simulink model "VSI"  (R2018b)
settings: Solver=FixedStepDiscrete  StartTime=0.0  StopTime=inf  FixedStep=0.01  RelTol=1e-3
PostLoadFcn:
  | if any(exist('dsrtsu_mdlpostloadfcn', 'file') ~= 0), dsrtsu_mdlpostloadfcn('Execute', bdroot); end
values from neighbouring files (symbols this model uses):
  d_WheelBase = 2.8    [VSI_Local.sldd]
  P_tARawFilt = 0.2    [VSI_Local.sldd]
  P_tAxsFilt = 0.2    [VSI_Local.sldd]
  P_tSasFilt = 0.25    [VSI_Local.sldd]
  P_tVVehFilt = 0.3    [VSI_Local.sldd]
  P_tYrsFilt = 0.25    [VSI_Local.sldd]
  P_vHi = 3.0    [VSI_Local.sldd]
  P_vLo = 1.0    [VSI_Local.sldd]
  StRatio = 15.2    [VSI_Local.sldd]
libraries: LPFilter x5
settings Model: DSRTSU_INTERNAL_RTI_VER=540  DSRTSU_INTERNAL_RTI_TYPE=rti1401  RTICANMMDATA=struct('GeneralSetupData',struct('modelroot','F:\DatabaseZO\08.Code\Model\ZOP_Integration','generalsettings',struct('filesettings',struct('destfolder',struct('Name','RTICANMM_FILES','Check',1),'buildfolder',struct('Name','.','Check',1),'AbsDestfolder',struct('Name','F:\DatabaseZO\08.Code\Model\ZOP_Integration\RTICANMM_FILES'),'AbsBuildfolder',struct('Name','F:\DatabaseZO\08.Code\Model\ZOP_Integration'))),'options',struct('addpaths',1,'rmpaths',1,'addtrcexclusion',logical(1),'cannavigator',struct('checkmonitoring',0),'show_usrtrc',0,'use_usrtrc',0),'advanced',struct('options',ones(1,100)),'MPSetup',{{}},'RTI',struct('Type','RTI1401','Ver','7.12','Date','02-May-2019'),'modelname','VSI','block','VSI'))  DSRTSU_INTERNAL_RTIFPGA=130  Creator=Administrator  LastModifiedBy=zjw
settings OptimizationCC: BlockReduction=off  ConditionallyExecuteInputs=off  OptimizeBlockIOStorage=off  BufferReuse=off  GlobalBufferReuse=off  ExpressionFolding=off  PassReuseOutputArgsThreshold=0  LocalBlockOutputs=off  OptimizeBlockOrder=speed  OptimizeDataStoreBuffers=off  BusAssignmentInplaceUpdate=off
settings DebuggingCC: ParameterTunabilityLossMsg=error
settings HardwareCC: ProdBitPerPointer=32  ProdBitPerSizeT=32  ProdBitPerPtrDiffT=32  ProdLargestAtomicInteger=Integer  ProdEndianess=BigEndian  ProdWordSize=32  ProdHWDeviceType=Custom Processor->Custom  TargetIntDivRoundTo=Zero  TargetEndianess=BigEndian  TargetHWDeviceType=Custom Processor->Custom
settings ModelReferenceCC: ModelReferenceNumInstancesAllowed=Single
settings SFSimCC: MATLABDynamicMemAlloc=off
settings RTWCC: SystemTargetFile=rti1401.tlc  MakeCommand=make_rti  TemplateMakefile=rti1401.tmf  Description=dSPACE DS1401 Hardware Platform  GenerateReport=on  LaunchReport=on
settings CodeAppCC: OperatorAnnotations=on
settings STFCustomTargetCC: ParMdlRefBuildCompliant=on  SystemTargetFile=rti1401.tlc
settings GRTTargetCC: TargetLangStandard=C89/C90 (ANSI)  CompOptLevelCompliant=off  ConcurrentExecutionCompliant=off  CombineOutputUpdateFcns=off  MatFileLogging=off  CPPClassGenCompliant=off  UseToolchainInfoCompliant=off

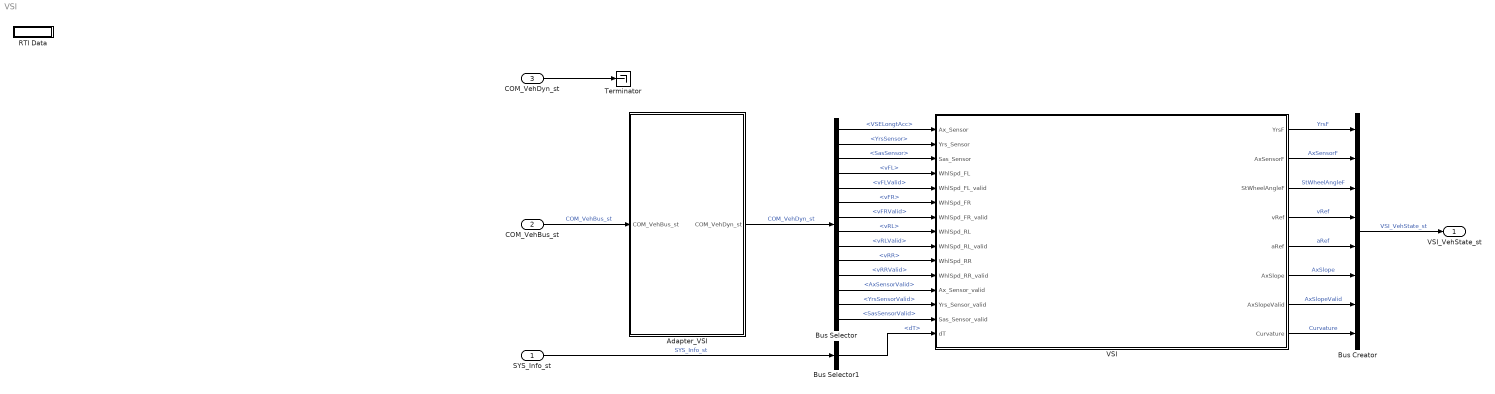
== system VSI ==
  SYS_Info_st : Inport  OutDataTypeStr=Bus: SYS_INFO_ST  BusOutputAsStruct=on
  COM_VehBus_st : Inport  Port=2  OutDataTypeStr=Bus: COM_VEHBUS_ST  BusOutputAsStruct=on
  COM_VehDyn_st : Inport  Port=3  OutDataTypeStr=Bus: COM_VEHDYN_ST  BusOutputAsStruct=on
  Adapter_VSI : Subsystem
  Bus Creator : BusCreator  Inputs=8  OutDataTypeStr=Bus: VSI_VEHSTATE_ST  NonVirtualBus=on
      settings: InheritFromInputs=off
  Bus Selector : BusSelector  OutputSignals=VSELongtAcc,YrsSensor,SasSensor,vFL,vFLValid,vFR,vFRValid,vRL,vRLValid,vRR,vRRValid,AxSensorValid,YrsSensorValid,SasSensorValid
  Bus Selector1 : BusSelector  OutputSignals=dT
  RTI Data : Subsystem  Tag=struct('RTIDataServer',struct('RTIDataServerVs','2','RTIModelDescription','struct(''main'',''VSI'',''sub'','''',''isMp'',0)'))  LoadFcn="if exist('rtidc'), try,  rtidc('DataHostBlockClbLoad', gcbh); catch, disp(['Warning: ''LoadFcn'' for RTI Data block failed: ' lasterr]); end, end,"  mask(RTI_DATA_HOST){}
      mask help:
      | RTI Data Block.
      | This block is used by RTI to store internal model-dependent data.
      | Please keep this block on the root level of the model. Deleting this block will result in data loss.
      |
      | NEVER DELETE OR COPY THIS BLOCK!
      settings: CopyFcn="if exist('rtidc'), try,  rtidc('DataHostBlockClbCopy', gcbh); catch, disp(['Warning: ''CopyFcn'' for RTI Data block failed: ' lasterr]); end, end,"  DeleteFcn="if exist('rtidc'), try,  rtidc('DataHostBlockClbDelete', gcbh); catch, disp(['Warning: ''DeleteFcn'' for RTI Data block failed: ' lasterr]); end, end,"  ModelCloseFcn="if exist('rtidc'), try,  rtidc('DataHostBlockClbModelClose', gcbh); catch, disp(['Warning: ''ModelCloseFcn'' for RTI Data block failed: ' lasterr]); end, end,"  PreSaveFcn="if exist('rtidc'), try,  rtidc('DataHostBlockClbPreSave', gcbh); catch, disp(['Warning: ''PreSaveFcn'' for RTI Data block failed: ' lasterr]); end, end,"  PostSaveFcn="if exist('rtidc'), try,  rtidc('DataHostBlockClbPostSave', gcbh); catch, disp(['Warning: ''PostSaveFcn'' for RTI Data block failed: ' lasterr]); end, end,"  NameChangeFcn="if exist('rtidc'), try,  rtidc('DataHostBlockClbNameChange', gcbh); catch, disp(['Warning: ''NameChangeFcn'' for RTI Data block failed: ' lasterr]); end, end,"
      mask Help:
      | RTI Data Block.
      | This block is used by RTI to store internal model-dependent data.
      | Please keep this block on the root level of the model. Deleting this block will result in data loss.
      | 
      | NEVER DELETE OR COPY THIS BLOCK!
      mask Display:
      | text(0.5, 0.5, 'RTI Data', 'HorizontalAlignment', 'center');
      | plot([1 0]);
  Terminator : Terminator
  VSI : Subsystem
  VSI_VehState_st : Outport  OutDataTypeStr=Bus: VSI_VEHSTATE_ST
  wires:
  Bus Selector/2 -> VSI/2(Yrs_Sensor)  "<YrsSensor>"
  Bus Selector/3 -> VSI/3(Sas_Sensor)  "<SasSensor>"
  Bus Selector/4 -> VSI/4(WhlSpd_FL)  "<vFL>"
  Bus Selector/5 -> VSI/5(WhlSpd_FL_valid)  "<vFLValid>"
  Bus Selector/6 -> VSI/6(WhlSpd_FR)  "<vFR>"
  Bus Selector/7 -> VSI/7(WhlSpd_FR_valid)  "<vFRValid>"
  Bus Selector/8 -> VSI/8(WhlSpd_RL)  "<vRL>"
  Bus Selector/9 -> VSI/9(WhlSpd_RL_valid)  "<vRLValid>"
  Bus Selector/10 -> VSI/10(WhlSpd_RR)  "<vRR>"
  Bus Selector/11 -> VSI/11(WhlSpd_RR_valid)  "<vRRValid>"
  Bus Selector/14 -> VSI/14(Sas_Sensor_valid)  "<SasSensorValid>"
  Bus Creator/1 -> VSI_VehState_st/1  "VSI_VehState_st"
  VSI/2(AxSensorF) -> Bus Creator/2  "AxSensorF"
  VSI/3(StWheelAngleF) -> Bus Creator/3  "StWheelAngleF"
  VSI/4(vRef) -> Bus Creator/4  "vRef"
  VSI/5(aRef) -> Bus Creator/5  "aRef"
  VSI/6(AxSlope) -> Bus Creator/6  "AxSlope"
  VSI/1(YrsF) -> Bus Creator/1  "YrsF"
  VSI/7(AxSlopeValid) -> Bus Creator/7  "AxSlopeValid"
  VSI/8(Curvature) -> Bus Creator/8  "Curvature"
  Bus Selector/12 -> VSI/12(Ax_Sensor_valid)  "<AxSensorValid>"
  Bus Selector/13 -> VSI/13(Yrs_Sensor_valid)  "<YrsSensorValid>"
  SYS_Info_st/1 -> Bus Selector1/1  "SYS_Info_st"
  Bus Selector1/1 -> VSI/15(dT)  "<dT>"
  COM_VehBus_st/1 -> Adapter_VSI/1(COM_VehBus_st)  "COM_VehBus_st"
  Bus Selector/1 -> VSI/1(Ax_Sensor)  "<VSELongtAcc>"
  Adapter_VSI/1(COM_VehDyn_st) -> Bus Selector/1  "COM_VehDyn_st"
  COM_VehDyn_st/1 -> Terminator/1

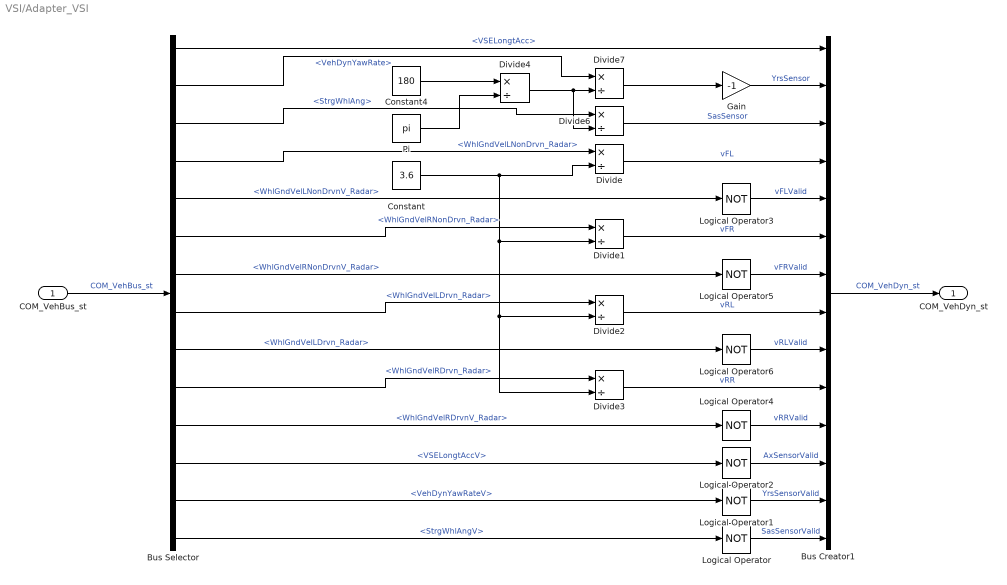
== system VSI/Adapter_VSI ==
  COM_VehBus_st : Inport  OutDataTypeStr=Bus: COM_VEHBUS_ST
  Bus Creator1 : BusCreator  Inputs=14  OutDataTypeStr=Bus: COM_VEHDYN_ST  NonVirtualBus=on
  Bus Selector : BusSelector  OutputSignals=x185.VSELongtAcc,x1E9.VehDynYawRate,x1E5.StrgWhlAng,x24E.WhlGndVelLNonDrvn_Radar,x24E.WhlGndVelLNonDrvnV_Radar,x24E.WhlGndVelRNonDrvn_Radar,x24E.WhlGndVelRNonDrvnV_Radar,x24C.WhlGndVelLDrvn_Radar,x24C.WhlGndVelLDrvn_Radar,x24C.WhlGndVelRDrvn_Radar,x24C.WhlGndVelRDrvnV_Radar,x185.VSELongtAccV,x1E9.VehDynYawRateV,x1E5.StrgWhlAngV
  Constant : Constant  Value=3.6
  Constant4 : Constant  Value=180
  Divide{,1..3,6..7} (6 alike) : Product  Inputs=*/  OutDataTypeStr=single
  Divide4 : Product  Inputs=*/
  Gain : Gain  Gain=-1
  Logical Operator{,1..6} (7 alike) : Logic  Operator=NOT  AllPortsSameDT=off  OutDataTypeStr=boolean
  Pi : Constant  Value=pi  OutDataTypeStr=Inherit: Inherit via back propagation
  COM_VehDyn_st : Outport  OutDataTypeStr=Bus: COM_VEHDYN_ST
  wires:
  Divide3/1 -> Bus Creator1/10  "vRR"
  Divide4/1 -> Divide6/2, Divide7/2
  Logical Operator2/1 -> Bus Creator1/12  "AxSensorValid"
  Divide/1 -> Bus Creator1/4  "vFL"
  Logical Operator1/1 -> Bus Creator1/13  "YrsSensorValid"
  Divide7/1 -> Gain/1
  Divide6/1 -> Bus Creator1/3  "SasSensor"
  Constant4/1 -> Divide4/1
  Logical Operator5/1 -> Bus Creator1/7  "vFRValid"
  Divide1/1 -> Bus Creator1/6  "vFR"
  Logical Operator4/1 -> Bus Creator1/11  "vRRValid"
  Bus Creator1/1 -> COM_VehDyn_st/1  "COM_VehDyn_st"
  Logical Operator3/1 -> Bus Creator1/5  "vFLValid"
  Divide2/1 -> Bus Creator1/8  "vRL"
  Logical Operator6/1 -> Bus Creator1/9  "vRLValid"
  Constant/1 -> Divide3/2, Divide2/2, Divide1/2, Divide/2
  Logical Operator/1 -> Bus Creator1/14  "SasSensorValid"
  COM_VehBus_st/1 -> Bus Selector/1  "COM_VehBus_st"
  Bus Selector/1 -> Bus Creator1/1  "<VSELongtAcc>"
  Pi/1 -> Divide4/2
  Bus Selector/2 -> Divide7/1  "<VehDynYawRate>"
  Bus Selector/5 -> Logical Operator3/1  "<WhlGndVelLNonDrvnV_Radar>"
  Bus Selector/7 -> Logical Operator5/1  "<WhlGndVelRNonDrvnV_Radar>"
  Bus Selector/9 -> Logical Operator6/1  "<WhlGndVelLDrvn_Radar>"
  Bus Selector/11 -> Logical Operator4/1  "<WhlGndVelRDrvnV_Radar>"
  Bus Selector/12 -> Logical Operator2/1  "<VSELongtAccV>"
  Bus Selector/13 -> Logical Operator1/1  "<VehDynYawRateV>"
  Bus Selector/14 -> Logical Operator/1  "<StrgWhlAngV>"
  Bus Selector/4 -> Divide/1  "<WhlGndVelLNonDrvn_Radar>"
  Bus Selector/6 -> Divide1/1  "<WhlGndVelRNonDrvn_Radar>"
  Bus Selector/8 -> Divide2/1  "<WhlGndVelLDrvn_Radar>"
  Bus Selector/10 -> Divide3/1  "<WhlGndVelRDrvn_Radar>"
  Bus Selector/3 -> Divide6/1  "<StrgWhlAng>"
  Gain/1 -> Bus Creator1/2  "YrsSensor"

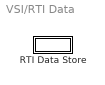
== system VSI/RTI Data ==
  RTI Data Store : Subsystem  Tag="struct('private',struct('version',struct('dsVer',uint32(2),'dsVerCreation',uint32(2),'RTI',struct('ver','7.12','type','RTI1401')),'access',struct('type','Model','isPerm',1,'created',['20-Nov-2020 11:10:38'],'modified',['07-Jan-2021 20:09:42'],'location','')),'public',struct('main',struct('data',[]),'sub',struct('name',{{'VSI'}},'data',{{struct('TH',struct('thTaskInfo',struct('taskType',{'TIMER','HWINT','TMRINT','SWINT','GLINT'},'tasksNumOf',{1,0,0,0,0},'srcIds',{{'TIMERA'},{},{},{},{}},'taskNames',{{['Timer Task 1']},{},{},{},{}})),'th_tc',struct('dataType','TASK','taskGroupId','','taskGroupList',{{}},'taskSchedulingPolicy','FCFS','taskType','TIMER','blkh',-1,'srcId','TIMERA','srcSgnName',['Timer A interrupt'],'srcCpuName','','taskName',['Timer Task 1  [0.01] s'],'taskNameDisplayExt','','smplTime',0.01,'smplTimeOffs',0,'hasFixedPriority',0,'priority',1,'hasFixedOvc',0,'ovcType',1,'ovcMax',1),'tc_th',struct('dataType','TASK','taskGroupId','','taskGroupList',{{}},'taskSchedulingPolicy','FCFS','taskType','TIMER','blkh',-1,'srcId','TIMERA','srcSgnName',['Timer A interrupt'],'srcCpuName','','taskName',['Timer Task 1  [0.01] s'],'taskNameDisplayExt','','smplTime',0.01,'smplTimeOffs',0,'hasFixedPriority',0,'priority',1,'hasFixedOvc',0,'ovcType',3,'ovcMax',1))}})))"  mask(RTI_DATA_STORE){}
      mask help:
      | RTI Data Store Block. This block is used by RTI to store internal model dependent data. Deleting this block will result in data loss.
      |
      | NEVER DELETE, COPY, OR MODIFY THIS BLOCK!
      mask Help:
      | RTI Data Store Block. This block is used by RTI to store internal model dependent data. Deleting this block will result in data loss.
      | 
      | NEVER DELETE, COPY, OR MODIFY THIS BLOCK!
      mask Display: text(0.5, 0.5, ' ', 'HorizontalAlignment', 'center');

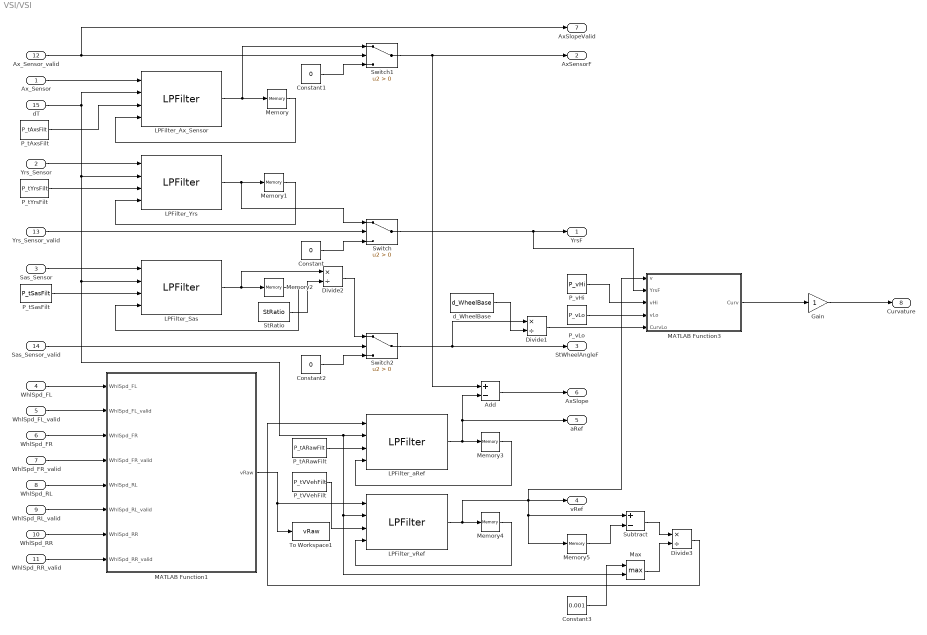
== system VSI/VSI ==
  Ax_Sensor : Inport
  Yrs_Sensor : Inport  Port=2
  Sas_Sensor : Inport  Port=3
  WhlSpd_FL : Inport  Port=4
  WhlSpd_FL_valid : Inport  Port=5
  WhlSpd_FR : Inport  Port=6
  WhlSpd_FR_valid : Inport  Port=7
  WhlSpd_RL : Inport  Port=8
  WhlSpd_RL_valid : Inport  Port=9
  WhlSpd_RR : Inport  Port=10
  WhlSpd_RR_valid : Inport  Port=11
  Ax_Sensor_valid : Inport  Port=12
  Yrs_Sensor_valid : Inport  Port=13
  Sas_Sensor_valid : Inport  Port=14
  dT : Inport  Port=15
  Add : Sum  Inputs=+-
  Constant : Constant  Value=0
  Constant1 : Constant  Value=0
  Constant2 : Constant  Value=0
  Constant3 : Constant  Value=0.001
  Divide1 : Product  Inputs=*/
  Divide2 : Product  Inputs=*/
  Divide3 : Product  Inputs=*/
  Gain : Gain
  LPFilter_Ax_Sensor : LPFilter/LPFilter  SystemSampleTime=-1
      settings: SourceProductName=CustomLib
  LPFilter_Sas : LPFilter/LPFilter  SystemSampleTime=-1
      settings: SourceProductName=CustomLib
  LPFilter_Yrs : LPFilter/LPFilter  SystemSampleTime=-1
      settings: SourceProductName=CustomLib
  LPFilter_aRef : LPFilter/LPFilter  SystemSampleTime=-1
      settings: SourceProductName=CustomLib
  LPFilter_vRef : LPFilter/LPFilter  SystemSampleTime=-1
      settings: SourceProductName=CustomLib
  MATLAB Function1 : MATLAB Function  TreatAsAtomicUnit=on
  MATLAB Function3 : MATLAB Function  TreatAsAtomicUnit=on
  Max : MinMax  Function=max  Inputs=2  OutDataTypeStr=single
  Memory{,1..5} (6 alike) : Memory
  P_tARawFilt : Constant  Value=P_tARawFilt
  P_tAxsFilt : Constant  Value=P_tAxsFilt
  P_tSasFilt : Constant  Value=P_tSasFilt
  P_tVVehFilt : Constant  Value=P_tVVehFilt
  P_tYrsFilt : Constant  Value=P_tYrsFilt
  P_vHi : Constant  Value=P_vHi
  P_vLo : Constant  Value=P_vLo
  StRatio : Constant  Value=StRatio
  Subtract : Sum  Inputs=+-
  Switch : Switch  Criteria=u2 > Threshold  OutDataTypeStr=single
  Switch1 : Switch  Criteria=u2 > Threshold  OutDataTypeStr=single
  Switch2 : Switch  Criteria=u2 > Threshold
  To Workspace1 : ToWorkspace  VariableName=vRaw  SaveFormat=Timeseries  SampleTime=-1
  d_WheelBase : Constant  Value=d_WheelBase
  YrsF : Outport
  AxSensorF : Outport  Port=2
  StWheelAngleF : Outport  Port=3
  vRef : Outport  Port=4
  aRef : Outport  Port=5
  AxSlope : Outport  Port=6
  AxSlopeValid : Outport  Port=7
  Curvature : Outport  Port=8
  wires:
  Switch1/1 -> AxSensorF/1, Add/1
  LPFilter_aRef/1 -> Memory3/1, aRef/1, Add/2
  Switch2/1 -> StWheelAngleF/1, Divide1/1
  WhlSpd_RR/1 -> MATLAB Function1/7(WhlSpd_RR)
  Constant2/1 -> Switch2/3
  MATLAB Function3/1(Curv) -> Gain/1
  MATLAB Function1/1(vRaw) -> To Workspace1/1, LPFilter_vRef/1
  WhlSpd_RL/1 -> MATLAB Function1/5(WhlSpd_RL)
  Switch/1 -> MATLAB Function3/2(YrsF), YrsF/1
  Constant/1 -> Switch/3
  Constant1/1 -> Switch1/3
  LPFilter_Ax_Sensor/1 -> Memory/1, Switch1/1
  P_vHi/1 -> MATLAB Function3/3(vHi)
  Ax_Sensor/1 -> LPFilter_Ax_Sensor/1
  Add/1 -> AxSlope/1
  Sas_Sensor_valid/1 -> Switch2/2
  WhlSpd_FL/1 -> MATLAB Function1/1(WhlSpd_FL)
  WhlSpd_FL_valid/1 -> MATLAB Function1/2(WhlSpd_FL_valid)
  WhlSpd_FR/1 -> MATLAB Function1/3(WhlSpd_FR)
  WhlSpd_FR_valid/1 -> MATLAB Function1/4(WhlSpd_FR_valid)
  WhlSpd_RL_valid/1 -> MATLAB Function1/6(WhlSpd_RL_valid)
  Yrs_Sensor_valid/1 -> Switch/2
  WhlSpd_RR_valid/1 -> MATLAB Function1/8(WhlSpd_RR_valid)
  Ax_Sensor_valid/1 -> AxSlopeValid/1, Switch1/2
  P_vLo/1 -> MATLAB Function3/4(vLo)
  Divide1/1 -> MATLAB Function3/5(CurvLo)
  dT/1 -> Max/2, LPFilter_vRef/2, LPFilter_aRef/2, LPFilter_Sas/2, LPFilter_Yrs/2, LPFilter_Ax_Sensor/2
  P_tAxsFilt/1 -> LPFilter_Ax_Sensor/3
  Yrs_Sensor/1 -> LPFilter_Yrs/1
  LPFilter_Yrs/1 -> Memory1/1, Switch/1
  P_tYrsFilt/1 -> LPFilter_Yrs/3
  LPFilter_Sas/1 -> Memory2/1, Divide2/1
  Sas_Sensor/1 -> LPFilter_Sas/1
  P_tSasFilt/1 -> LPFilter_Sas/3
  Divide2/1 -> Switch2/1
  StRatio/1 -> Divide2/2
  P_tARawFilt/1 -> LPFilter_aRef/3
  LPFilter_vRef/1 -> Memory4/1, MATLAB Function3/1(v), Memory5/1, Subtract/1, vRef/1
  P_tVVehFilt/1 -> LPFilter_vRef/3
  Memory5/1 -> Subtract/2
  Divide3/1 -> LPFilter_aRef/1
  Subtract/1 -> Divide3/1
  Memory3/1 -> LPFilter_aRef/4
  Memory4/1 -> LPFilter_vRef/4
  Memory/1 -> LPFilter_Ax_Sensor/4
  Memory1/1 -> LPFilter_Yrs/4
  Memory2/1 -> LPFilter_Sas/4
  Max/1 -> Divide3/2
  Constant3/1 -> Max/1
  d_WheelBase/1 -> Divide1/2
  Gain/1 -> Curvature/1

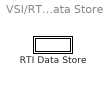
== system VSI/RTI Data/RTI Data Store ==
  RTI Data Store : Subsystem  mask(RTI_DATA_STORE){}
      mask help:
      | RTI Data Store Block. This block is used by RTI to store internal model dependent data. Deleting this block will result in data loss.
      |
      | NEVER DELETE, COPY, OR MODIFY THIS BLOCK!
      mask Help:
      | RTI Data Store Block. This block is used by RTI to store internal model dependent data. Deleting this block will result in data loss.
      | 
      | NEVER DELETE, COPY, OR MODIFY THIS BLOCK!
      mask Display: text(0.5, 0.5, ' ', 'HorizontalAlignment', 'center');

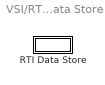
== system VSI/RTI Data/RTI Data Store/RTI Data Store ==
  RTI Data Store : Subsystem  mask(RTI_DATA_STORE){}
      mask help:
      | RTI Data Store Block. This block is used by RTI to store internal model dependent data. Deleting this block will result in data loss.
      |
      | NEVER DELETE, COPY, OR MODIFY THIS BLOCK!
      mask Help:
      | RTI Data Store Block. This block is used by RTI to store internal model dependent data. Deleting this block will result in data loss.
      | 
      | NEVER DELETE, COPY, OR MODIFY THIS BLOCK!
      mask Display: text(0.5, 0.5, ' ', 'HorizontalAlignment', 'center');

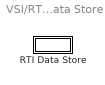
== system VSI/RTI Data/RTI Data Store/RTI Data Store/RTI Data Store ==
  RTI Data Store : Subsystem  mask(RTI_DATA_STORE){}
      mask help:
      | RTI Data Store Block. This block is used by RTI to store internal model dependent data. Deleting this block will result in data loss.
      |
      | NEVER DELETE, COPY, OR MODIFY THIS BLOCK!
      mask Help:
      | RTI Data Store Block. This block is used by RTI to store internal model dependent data. Deleting this block will result in data loss.
      | 
      | NEVER DELETE, COPY, OR MODIFY THIS BLOCK!
      mask Display: text(0.5, 0.5, ' ', 'HorizontalAlignment', 'center');

== system VSI/RTI Data/RTI Data Store/RTI Data Store/RTI Data Store/RTI Data Store ==

== matlab function VSI/MATLAB Function1 ==
  data: WhlSpd_FL input; WhlSpd_FL_valid input; WhlSpd_FR input; WhlSpd_FR_valid input; WhlSpd_RL input; WhlSpd_RL_valid input; WhlSpd_RR input; WhlSpd_RR_valid input; vRaw output
function vRaw = vRef_cal(WhlSpd_FL,WhlSpd_FL_valid,WhlSpd_FR,WhlSpd_FR_valid,WhlSpd_RL,WhlSpd_RL_valid,WhlSpd_RR,WhlSpd_RR_valid)

WhlSpd_valid_cnt = 0;
if (WhlSpd_FL_valid)
    WhlSpd_valid_cnt = WhlSpd_valid_cnt + 1;
else
end
if (WhlSpd_FR_valid)
    WhlSpd_valid_cnt = WhlSpd_valid_cnt + 1;
else
end
if (WhlSpd_RL_valid)
    WhlSpd_valid_cnt = WhlSpd_valid_cnt + 1;
else
end
if (WhlSpd_RR_valid)
    WhlSpd_valid_cnt = WhlSpd_valid_cnt + 1;
else
end

if (WhlSpd_valid_cnt == 4)
    v_FA = (WhlSpd_FL + WhlSpd_FR)/2;
    v_RA = (WhlSpd_RL + WhlSpd_RR)/2;
if (v_FA >= v_RA)
    vRaw = (min(WhlSpd_FL,WhlSpd_FR)+max(WhlSpd_RL,WhlSpd_RR))/2;
else
    vRaw = (max(WhlSpd_FL,WhlSpd_FR)+min(WhlSpd_RL,WhlSpd_RR))/2;
end
else
    vRaw = (WhlSpd_FL * WhlSpd_FL_valid + WhlSpd_FR * WhlSpd_FR_valid + WhlSpd_RL * WhlSpd_RL_valid + WhlSpd_RR * WhlSpd_RR_valid)/WhlSpd_valid_cnt;
end

== matlab function VSI/MATLAB Function3 ==
  data: v input; YrsF input; Curv output; vHi input; vLo input; CurvLo input
function Curv = Curvature(v,YrsF,vHi,vLo,CurvLo)

if (v < vLo)
    Curv = CurvLo;
elseif (v > vHi)
    Curv = YrsF/v;
else
    Curv = (v - vLo)/(vHi - vLo)*(YrsF/v - CurvLo) + CurvLo;
end
